simulink library "Tools_6dofSimulation"  (R2018a)
settings: Solver=VariableStepAuto  StartTime=0.0  StopTime=10.0  RelTol=1e-3
libraries: sharedutil x3
settings Model: Creator=abhineet  LastModifiedBy=abhineet

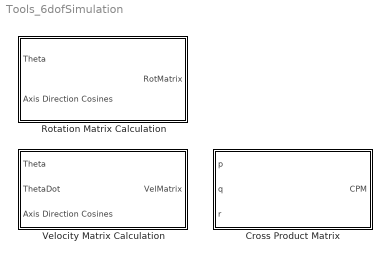
== system Tools_6dofSimulation ==
  Cross Product Matrix : Subsystem
  Rotation Matrix Calculation : Subsystem
  Velocity Matrix Calculation : Subsystem

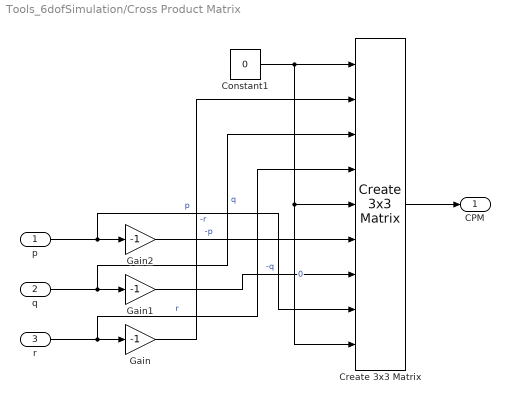
== system Tools_6dofSimulation/Cross Product Matrix ==
  p : Inport
  q : Inport  Port=2
  r : Inport  Port=3
  Constant1 : Constant  Value=0
  Create 3x3 Matrix : sharedutil/Create 3x3 Matrix  aMode=aMode
  Gain : Gain  Gain=-1
  Gain1 : Gain  Gain=-1
  Gain2 : Gain  Gain=-1
  CPM : Outport
  wires:
  q/1 -> Create 3x3 Matrix/3, Gain1/1  "q"
  Gain/1 -> Create 3x3 Matrix/2  "-r"
  Gain2/1 -> Create 3x3 Matrix/6  "-p"
  Gain1/1 -> Create 3x3 Matrix/7  "-q"
  p/1 -> Create 3x3 Matrix/8, Gain2/1  "p"
  Create 3x3 Matrix/1 -> CPM/1
  Constant1/1 -> Create 3x3 Matrix/9, Create 3x3 Matrix/5, Create 3x3 Matrix/1  "0"
  r/1 -> Create 3x3 Matrix/4, Gain/1  "r"

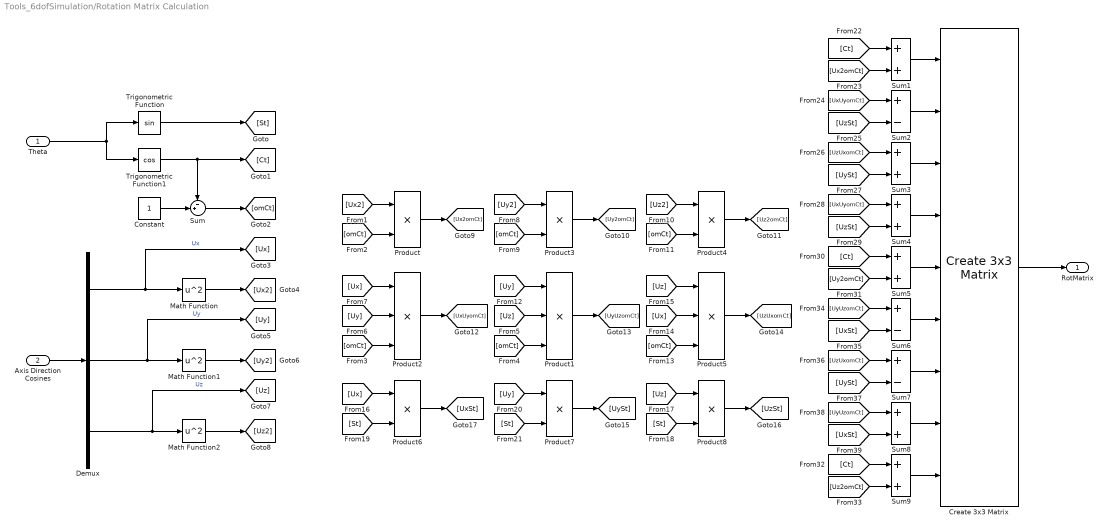
== system Tools_6dofSimulation/Rotation Matrix Calculation ==
  Theta : Inport
  Axis Direction Cosines : Inport  Port=2
  Constant : Constant
  Create 3x3 Matrix : sharedutil/Create 3x3 Matrix  aMode=aMode
  Demux : Demux  Outputs=3
  Math Function : Math  Operator=square  SaturateOnIntegerOverflow=on
  Math Function1 : Math  Operator=square  SaturateOnIntegerOverflow=on
  Math Function2 : Math  Operator=square  SaturateOnIntegerOverflow=on
  Product{,3..4,6..8} (6 alike) : Product
  Product1 : Product  Inputs=3
  Product2 : Product  Inputs=3
  Product5 : Product  Inputs=3
  Sum : Sum  Inputs=-+|
  Sum{1,3..5,8..9} (6 alike) : Sum
  Sum2 : Sum  Inputs=+-
  Sum6 : Sum  Inputs=+-
  Sum7 : Sum  Inputs=+-
  Trigonometric Function : Trigonometry
  Trigonometric Function1 : Trigonometry  Operator=cos
  RotMatrix : Outport
  wires:
  [omCt] -> Product3/2
  [St] -> Product8/2
  [omCt] -> Product/2
  [omCt] -> Product4/2
  [UxUyomCt] -> Sum4/1
  [Ct] -> Sum9/1
  [St] -> Product6/2
  [Ct] -> Sum5/1
  Product3/1 -> [Uy2omCt]
  [Ct] -> Sum1/1
  Product6/1 -> [UxSt]
  Sum2/1 -> Create 3x3 Matrix/2
  Product/1 -> [Ux2omCt]
  [Uz] -> Product8/1
  Trigonometric Function/1 -> [St]
  [Uy2] -> Product3/1
  Sum4/1 -> Create 3x3 Matrix/4
  Product8/1 -> [UzSt]
  [Uz2] -> Product4/1
  [omCt] -> Product5/3
  [omCt] -> Product2/3
  [UxSt] -> Sum6/2
  Product2/1 -> [UxUyomCt]
  Sum5/1 -> Create 3x3 Matrix/5
  [Ux] -> Product5/2
  Sum9/1 -> Create 3x3 Matrix/9
  [Ux2] -> Product/1
  Product4/1 -> [Uz2omCt]
  [UyUzomCt] -> Sum8/1
  Product5/1 -> [UzUxomCt]
  Demux/1 -> [Ux], Math Function/1  "Ux"
  Axis Direction Cosines/1 -> Demux/1
  Demux/2 -> [Uy], Math Function1/1  "Uy"
  Product7/1 -> [UySt]
  [Uy] -> Product1/1
  Create 3x3 Matrix/1 -> RotMatrix/1
  Theta/1 -> Trigonometric Function/1, Trigonometric Function1/1
  Math Function1/1 -> [Uy2]
  Math Function2/1 -> [Uz2]
  Math Function/1 -> [Ux2]
  [Uy2omCt] -> Sum5/2
  [UySt] -> Sum3/2
  [omCt] -> Product1/3
  [St] -> Product7/2
  Sum3/1 -> Create 3x3 Matrix/3
  [Ux] -> Product6/1
  Sum8/1 -> Create 3x3 Matrix/8
  [UySt] -> Sum7/2
  Demux/3 -> [Uz], Math Function2/1  "Uz"
  [Uz] -> Product5/1
  [UzSt] -> Sum4/2
  [UyUzomCt] -> Sum6/1
  [Uz] -> Product1/2
  [Uy] -> Product2/2
  [Ux] -> Product2/1
  Sum7/1 -> Create 3x3 Matrix/7
  Sum1/1 -> Create 3x3 Matrix/1
  Constant/1 -> Sum/2
  Product1/1 -> [UyUzomCt]
  Trigonometric Function1/1 -> Sum/1, [Ct]
  Sum6/1 -> Create 3x3 Matrix/6
  [UzUxomCt] -> Sum7/1
  [UxUyomCt] -> Sum2/1
  [UzSt] -> Sum2/2
  [Uz2omCt] -> Sum9/2
  Sum/1 -> [omCt]
  [UxSt] -> Sum8/2
  [Ux2omCt] -> Sum1/2
  [Uy] -> Product7/1
  [UzUxomCt] -> Sum3/1

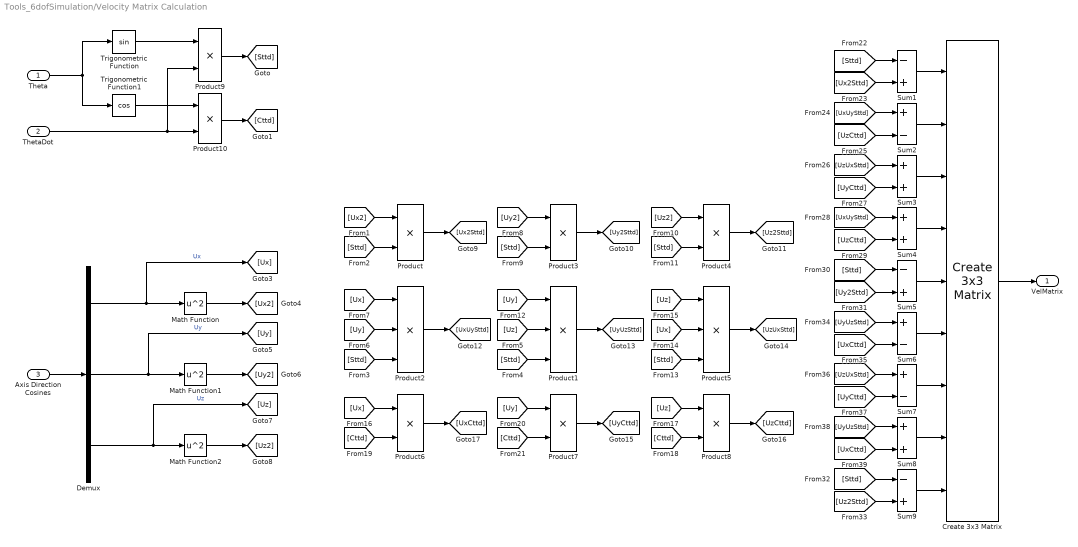
== system Tools_6dofSimulation/Velocity Matrix Calculation ==
  Theta : Inport
  ThetaDot : Inport  Port=2
  Axis Direction Cosines : Inport  Port=3
  Create 3x3 Matrix : sharedutil/Create 3x3 Matrix  aMode=aMode
  Demux : Demux  Outputs=3
  Math Function : Math  Operator=square  SaturateOnIntegerOverflow=on
  Math Function1 : Math  Operator=square  SaturateOnIntegerOverflow=on
  Math Function2 : Math  Operator=square  SaturateOnIntegerOverflow=on
  Product{,3..4,6..10} (8 alike) : Product
  Product1 : Product  Inputs=3
  Product2 : Product  Inputs=3
  Product5 : Product  Inputs=3
  Sum1 : Sum  Inputs=-+
  Sum2 : Sum  Inputs=+-
  Sum3 : Sum
  Sum4 : Sum
  Sum5 : Sum  Inputs=-+
  Sum6 : Sum  Inputs=+-
  Sum7 : Sum  Inputs=+-
  Sum8 : Sum
  Sum9 : Sum  Inputs=-+
  Trigonometric Function : Trigonometry
  Trigonometric Function1 : Trigonometry  Operator=cos
  VelMatrix : Outport
  wires:
  Product2/1 -> [UxUySttd]
  [UxCttd] -> Sum6/2
  [UxUySttd] -> Sum4/1
  [UzUxSttd] -> Sum7/1
  [UzUxSttd] -> Sum3/1
  [Sttd] -> Product/2
  Sum9/1 -> Create 3x3 Matrix/9
  [Sttd] -> Product3/2
  [Ux2Sttd] -> Sum1/2
  Product/1 -> [Ux2Sttd]
  [Ux] -> Product6/1
  Product8/1 -> [UzCttd]
  [Cttd] -> Product7/2
  [Uy2] -> Product3/1
  [Sttd] -> Sum5/1
  Sum2/1 -> Create 3x3 Matrix/2
  [UxCttd] -> Sum8/2
  [Cttd] -> Product8/2
  [Uy] -> Product7/1
  [Uz] -> Product8/1
  [Uz2Sttd] -> Sum9/2
  [Sttd] -> Sum1/1
  Product7/1 -> [UyCttd]
  Create 3x3 Matrix/1 -> VelMatrix/1
  [UyCttd] -> Sum3/2
  [Cttd] -> Product6/2
  [Sttd] -> Product2/3
  Demux/3 -> [Uz], Math Function2/1  "Uz"
  [UzCttd] -> Sum2/2
  Sum4/1 -> Create 3x3 Matrix/4
  Sum3/1 -> Create 3x3 Matrix/3
  [Uy] -> Product1/1
  [Uz2] -> Product4/1
  Sum8/1 -> Create 3x3 Matrix/8
  Product6/1 -> [UxCttd]
  Product3/1 -> [Uy2Sttd]
  [UyUzSttd] -> Sum6/1
  Demux/1 -> [Ux], Math Function/1  "Ux"
  [UxUySttd] -> Sum2/1
  [Ux] -> Product5/2
  Sum1/1 -> Create 3x3 Matrix/1
  Axis Direction Cosines/1 -> Demux/1
  Sum6/1 -> Create 3x3 Matrix/6
  Sum5/1 -> Create 3x3 Matrix/5
  Math Function1/1 -> [Uy2]
  [Sttd] -> Sum9/1
  Sum7/1 -> Create 3x3 Matrix/7
  Product1/1 -> [UyUzSttd]
  [UyCttd] -> Sum7/2
  [Ux] -> Product2/1
  [UzCttd] -> Sum4/2
  Product4/1 -> [Uz2Sttd]
  [Sttd] -> Product5/3
  [Uz] -> Product1/2
  Product5/1 -> [UzUxSttd]
  [UyUzSttd] -> Sum8/1
  Demux/2 -> [Uy], Math Function1/1  "Uy"
  [Sttd] -> Product4/2
  Theta/1 -> Trigonometric Function/1, Trigonometric Function1/1
  [Ux2] -> Product/1
  Math Function2/1 -> [Uz2]
  [Uy2Sttd] -> Sum5/2
  Math Function/1 -> [Ux2]
  [Uz] -> Product5/1
  [Sttd] -> Product1/3
  [Uy] -> Product2/2
  Trigonometric Function/1 -> Product9/1
  Trigonometric Function1/1 -> Product10/1
  Product10/1 -> [Cttd]
  Product9/1 -> [Sttd]
  ThetaDot/1 -> Product9/2, Product10/2
